simulink model "simulation2"  (R2014b)
settings: Solver=ode45  StartTime=0.0  StopTime=400  RelTol=1e-3
libraries: simulink x1
settings Model: Creator=jonas  LastModifiedBy=jonas
settings DataIOCC: LimitDataPoints=off

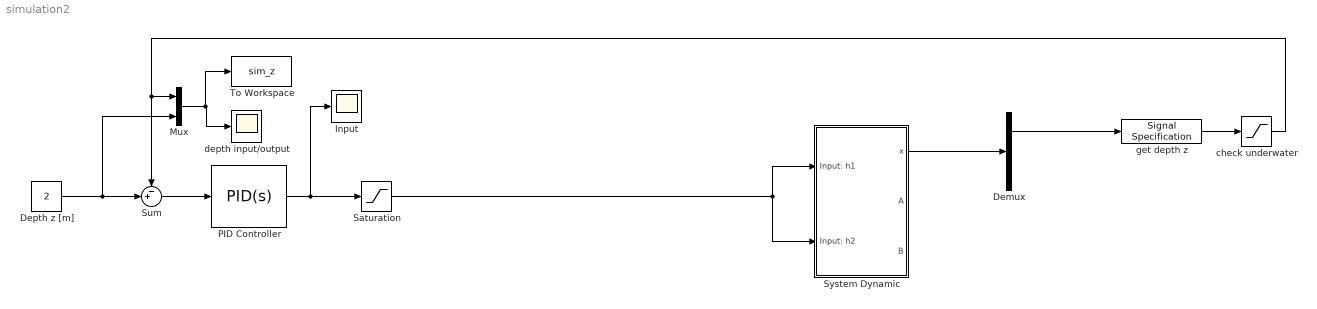
== system simulation2 ==
  Demux : Demux  Outputs=2
  Depth z [m] : Constant  Value=2
  Input : Scope
      settings: SaveName=ScopeData2
  Mux : Mux  Inputs=2
  PID Controller : simulink/Continuous/PID Controller  Controller=PID  TimeDomain=Continuous-time  SampleTime=-1  IntegratorMethod=Forward Euler  FilterMethod=Forward Euler  Form=Parallel  P=4.2637521462458  I=0.0940371071083085  D=7.66298301921273  N=2.63026799189538  InitialConditionSource=internal  InitialConditionForIntegrator=0  InitialConditionForFilter=0  ExternalReset=none  LimitOutput=on  UpperSaturationLimit=1  LowerSaturationLimit=0  LinearizeAsGain=on  AntiWindupMode=none  Kb=1  TrackingMode=off  Kt=1  PParamMin=[]  PParamMax=[]  IParamMin=[]  IParamMax=[]  DParamMin=[]  DParamMax=[]  NParamMin=[]  NParamMax=[]  KbParamMin=[]  KbParamMax=[]  KtParamMin=[]  KtParamMax=[]  POutMin=[]  POutMax=[]  IOutMin=[]  IOutMax=[]  DOutMin=[]  DOutMax=[]  NOutMin=[]  NOutMax=[]  KbOutMin=[]  KbOutMax=[]  KtOutMin=[]  KtOutMax=[]  IntegratorOutMin=[]  IntegratorOutMax=[]  FilterOutMin=[]  FilterOutMax=[]  SumOutMin=[]  SumOutMax=[]  SumI1OutMin=[]  SumI1OutMax=[]  SumI2OutMin=[]  SumI2OutMax=[]  SumI3OutMin=[]  SumI3OutMax=[]  SumDOutMin=[]  SumDOutMax=[]  SaturationOutMin=[]  SaturationOutMax=[]  IntegratorContinuousStateAttributes=''  IntegratorStateMustResolveToSignalObject=off  IntegratorRTWStateStorageClass=Auto  FilterContinuousStateAttributes=''  FilterStateMustResolveToSignalObject=off  FilterRTWStateStorageClass=Auto  DifferentiatorICPrevScaledInput=0  DifferentiatorOutMin=[]  DifferentiatorOutMax=[]  UseFilter=on
  Saturation : Saturate  UpperLimit=1  LowerLimit=0
  Sum : Sum  Inputs=-+|
  System Dynamic : Subsystem
  To Workspace : ToWorkspace  VariableName=sim_z  SampleTime=0.01
  check underwater : Saturate  UpperLimit=1000  LowerLimit=0
  depth input/output : Scope
      settings: SaveName=ScopeData3
  get depth z : SignalSpecification  Dimensions=1
  wires:
  get depth z/1 -> check underwater/1
  PID Controller/1 -> Input/1, Saturation/1
  Sum/1 -> PID Controller/1
  Mux/1 -> To Workspace/1, depth input/output/1
  Depth z [m]/1 -> Mux/2, Sum/2
  check underwater/1 -> Mux/1, Sum/1
  System Dynamic/1(x) -> Demux/1
  Demux/1 -> get depth z/1
  Saturation/1 -> System Dynamic/1(Input: h1), System Dynamic/2(Input: h2)

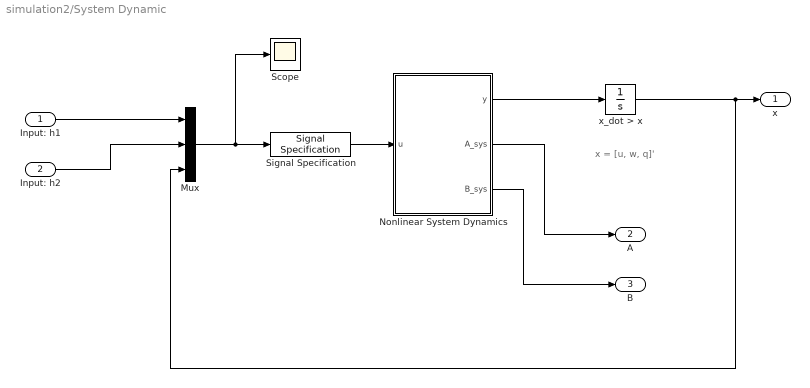
== system simulation2/System Dynamic ==
  note: x = [u, w, q]'
  Input: h1 : Inport
  Input: h2 : Inport  Port=2
  Mux : Mux  Inputs=3
  Nonlinear System Dynamics : MATLAB Function  TreatAsAtomicUnit=on
  Scope : Scope
      settings: SaveName=ScopeData4
  Signal Specification : SignalSpecification  Dimensions=10
  x_dot > x : Integrator
  x : Outport
  A : Outport  Port=2
  B : Outport  Port=3
  wires:
  Mux/1 -> Scope/1, Signal Specification/1
  Signal Specification/1 -> Nonlinear System Dynamics/1(u)
  x_dot > x/1 -> Mux/3, x/1
  Nonlinear System Dynamics/1(y) -> x_dot > x/1
  Input: h1/1 -> Mux/1
  Input: h2/1 -> Mux/2
  Nonlinear System Dynamics/2(A_sys) -> A/1
  Nonlinear System Dynamics/3(B_sys) -> B/1

== matlab function simulation2/System Dynamic/Nonlinear System Dynamics ==
  data: u input; y output; A_sys output; B_sys output
function [y,A_sys, B_sys] = fcn(u)
%#codegen

% ---- PARAMETERS ----

g   = 9.81;                 % [m/s^2]   gravity
rho = 1000;                 % [kg/m^3]  density water

% parameters nanins specific
m0  = 5.7;                    % [kg]      empty weight Nanin
l_n = 0.514;                  % [m]       length Nanin
r_n = 0.06;                  % [m]       radius Nanin
V_n = r_n^2*pi*l_n;         % [m^3]     volume Nanin

x0_t = 0.25;                % [m]       displacement piston tank in x direction
z0_t = 0.05;                % [m]       displacement piston tank in z direction
A_t = pi*(65/(2*1000))^2;   % [m^2]     area piston tank
V_t = 250e-6;               % [m^3]     volume of piston tank
h_max = V_t/A_t;            % [m]       max height of water in piston tank

Iy0 = 0.134;                % [kgm^2]   moment of inertia around y-axis

% restoring static forces
W_r = m0*g;          % [N]       gravitational force empty
B_r = rho*g*V_n;    % [N]       buoancy restoring force

% Added mass coefficents
Z_w = -rho*V_n;             % [kg]
M_q = -1/12*rho*V_n*l_n;    % [km*m]

% ------

% rename parameters for clarification
h1 = u(1);
h2 = u(2);
theta = u(4);
x = u(3:end);

% Denormalize input
h1 = h1*h_max;
h2 = h2*h_max;

u_sys = [h1, h2]';

% calculate dynamic parameters
m = m0 + rho*A_t*(h1+h2); % dynamic mass
x1 = x0_t - h1/2;         % CoG of piston tank
x2 = -(x0_t - h2/2);
X_u = -0.1*m;

z_g = 0.005;
x_g = 0;
I_y = Iy0;

% calculate system model matrices
M = [m-X_u, 0,      m*z_g;...
     0,     m-Z_w,  -m*x_g;...
     m*z_g, -m*x_g, I_y-M_q];
 
g_static = [(W_r-B_r)*sin(theta);...
            -(W_r-B_r)*cos(theta);...
            z_g*W_r*sin(theta) + x_g*W_r*cos(theta)];
        
G_dyn = g*rho*A_t*[sin(theta),  sin(theta);...
                    -cos(theta), -cos(theta);...
                    sin(theta)*z0_t+cos(theta)*x1, sin(theta)*z0_t+cos(theta)*x2];
                
% state x = [z theta u w q fu fw fq]
x(6:8) = g_static; % update state

M_inv = inv(M);

A = [zeros(2,2), [-sin(theta) cos(theta) 0; 0 0 1], zeros(2,3);...
    zeros(3,5), -M_inv;...
    zeros(3,8)];

B = [zeros(2,2);...
    -M_inv*G_dyn;...
    zeros(3,2)];

x_dot = A*x+B*u_sys;

% return values
y = x_dot;
A_sys = A;
B_sys = B;
